simulink model "SolarMPPTController_New"  (R2019b)
settings: Solver=FixedStepAuto  StartTime=0.0  StopTime=6.0  RelTol=1e-3
libraries: powerlib x9, re_lib x1, powerlib_meascontrol x1, simulink x1
settings Model: Creator=DELL  LastModifiedBy=DELL

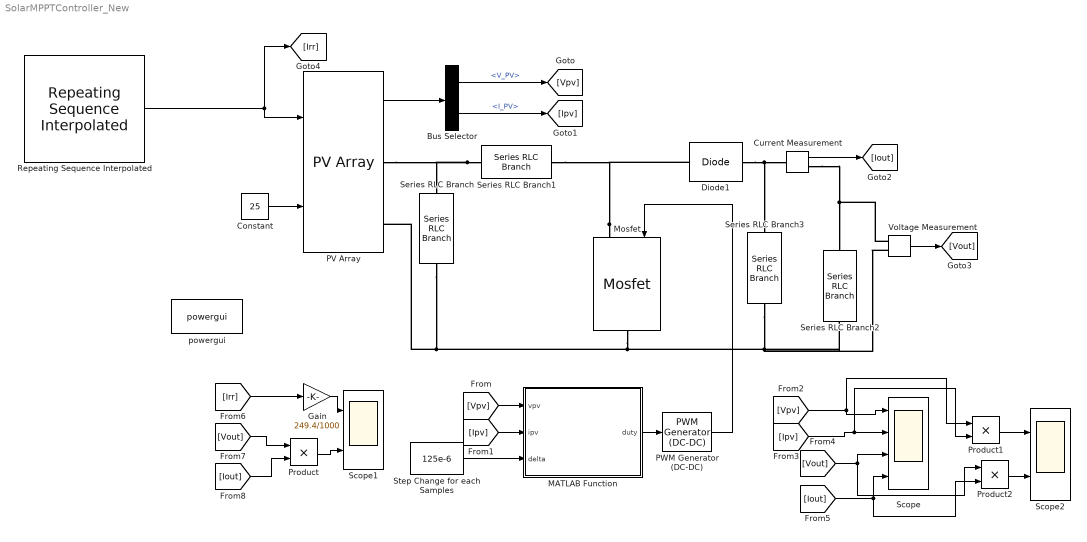
== system SolarMPPTController_New ==
  Bus Selector : BusSelector  OutputSignals=V_PV,I_PV
  Constant : Constant  Value=25
  Current Measurement : powerlib/Measurements/Current Measurement  PhasorSimulation=off  OutputType=Complex  PSBequivalent=0
      settings: SourceProductName=Simscape Electrical
  Diode1 : powerlib/Power Electronics/Diode  Ron=0.001  Lon=0  Vf=0.8  IC=0  UseSnubber=0  Rs=500  Cs=250e-9  Measurements=off
      settings: SourceProductName=Simscape Electrical
  Gain : Gain  Gain=249.4/1000
  MATLAB Function : MATLAB Function  TreatAsAtomicUnit=on
  Mosfet : powerlib/Power Electronics/Mosfet  Ron=0.1  Lon=0  Rd=0.01  Vfd=0  IC=0  Rs=1e5  Cs=inf  Measurements=off
      settings: SourceProductName=Simscape Electrical
  PV Array : re_lib/Solar/PV Array  Npar=1  Nser=1  PlotType=array @ 25 deg.C & specified irradiances  S_vec="[ 1000  500  100 ]"  Temp_C_vec="[ 45 25  ]"  ModuleName=1Soltech 1STH-FRL-4H-250-M60-BLK  PlotWhenSelected=off  Pm=248.977  Ncell=60  Voc=38.4  Isc=8.85  Vm=30.7  Im=8.11  beta_Voc_pc=-0.35599  alpha_Isc_pc=0.07  beta_Voc=-0.1367  alpha_Isc=0.006195  IL=8.8816  I0=2.622e-10  nI=1.0292  Rsh=104.8951  Rs=0.37421  BAL=off  Tc=1e-6  Tfilter=5e-5
      settings: SourceProductName=Simscape Electrical
  PWM Generator (DC-DC) : powerlib_meascontrol/Pulse & Signal Generators/PWM Generator (DC-DC)  Fsw=5000  Ts=1e-6
      settings: SourceProductName=Simscape Electrical
  Product : Product
  Product1 : Product
  Product2 : Product
  Repeating Sequence Interpolated : simulink/Sources/Repeating Sequence Interpolated  OutValues=[0 0 500 500 800 800 1000 1000 500 500 0 0]  TimeValues=[0 1.0 1.001 2.0 2.001 3.0 3.001 4.0 4.001 5.0 5.01 6.0]  LookUpMeth=Interpolation-Use End Values  tsamp=0.01  OutMin=[]  OutMax=[]  OutDataTypeStr=double  OutputDataTypeScalingMode=double  OutDataType=fixdt(0,8)  OutScaling=2^-10
  Scope : Scope  NumInputPorts=4
  Scope1 : Scope  NumInputPorts=2
  Scope2 : Scope  NumInputPorts=2
  Series RLC Branch : powerlib/Elements/Series RLC Branch  LConnTagsString=__new0  RConnTagsString=__new0  BranchType=C  Resistance=1e-6  Inductance=0  SetiL0=off  InitialCurrent=0  Capacitance=100e-6  Setx0=off  InitialVoltage=0  Measurements=None
      settings: SourceProductName=Simscape Electrical
  Series RLC Branch1 : powerlib/Elements/Series RLC Branch  LConnTagsString=__new0  RConnTagsString=__new0  BranchType=RL  Resistance=0.001  Inductance=900e-6  SetiL0=off  InitialCurrent=0  Capacitance=100e-6  Setx0=off  InitialVoltage=0  Measurements=None
      settings: SourceProductName=Simscape Electrical
  Series RLC Branch2 : powerlib/Elements/Series RLC Branch  LConnTagsString=__new0  RConnTagsString=__new0  BranchType=R  Resistance=20  Inductance=1e-3  SetiL0=off  InitialCurrent=0  Capacitance=100e-6  Setx0=off  InitialVoltage=0  Measurements=None
      settings: SourceProductName=Simscape Electrical
  Series RLC Branch3 : powerlib/Elements/Series RLC Branch  LConnTagsString=__new0  RConnTagsString=__new0  BranchType=C  Resistance=1e-6  Inductance=0  SetiL0=off  InitialCurrent=0  Capacitance=813e-6  Setx0=off  InitialVoltage=0  Measurements=None
      settings: SourceProductName=Simscape Electrical
  Step Change for each Samples : Constant  Value=125e-6
  Voltage Measurement : powerlib/Measurements/Voltage Measurement  PhasorSimulation=off  OutputType=Complex  PSBequivalent=0
      settings: SourceProductName=Simscape Electrical
  powergui : powerlib/powergui  Priority=1  SimulationMode=Discrete  SampleTime=5e-6  frequency=60  Iterations=50  frequencyindice=0  Pbase=100e6  ErrMax=1e-4  UnitsV=kV  UnitsW=MW  buscounter=0  FunctionMessages=off  echomessages=off  EnableUseOfTLC=off  CurrentSourceSwitches=off  DisableSnubberDevices=off  DisableRonSwitches=off  DisableVfSwitches=off  DisplayEquations=off  AutomaticDiscreteSolvers=off  SolverType=Tustin/Backward Euler (TBE)  Interpol=off  ExternalGateDelay=off  methode=off  Ts=100  x0status=blocks  SPID=on  SwTol=0  HookPort=off  NonlinearTolerance=1e-4  nMaxIteration=100  ContinueOnMaxIteration=off  RestoreLinks=warning  ResistiveCurrentMeasurement=off  Frange=[0:2:500]  Ylog=off  Xlog=on  ShowGrid=off  save=off  variable=ZData  structure=0  ZoomFFT=off  StartTime=0.0  cycles=1  DisplayStyle=1  fundamental=60  FreqAxis=off  MaxFrequency=1000  frequencyindicesteady=1  RmsSteady=1  display=off
      settings: SourceProductName=Simscape Electrical
  wires:
  Voltage Measurement/1 -> [Vout]
  [Ipv] -> Product1/2, Scope/2
  Step Change for each Samples/1 -> MATLAB Function/3(delta)
  [Vpv] -> Product1/1, Scope/1
  [Ipv] -> MATLAB Function/2(ipv)
  [Iout] -> Scope/4, Product2/2
  PV Array/1 -> Bus Selector/1
  MATLAB Function/1(duty) -> PWM Generator (DC-DC)/1
  PWM Generator (DC-DC)/1 -> Mosfet/1
  Bus Selector/2 -> [Ipv]  "<I_PV>"
  [Vpv] -> MATLAB Function/1(vpv)
  Bus Selector/1 -> [Vpv]  "<V_PV>"
  Constant/1 -> PV Array/2
  [Vout] -> Scope/3, Product2/1
  Current Measurement/1 -> [Iout]
  Repeating Sequence Interpolated/1 -> PV Array/1, [Irr]
  [Irr] -> Gain/1
  Gain/1 -> Scope1/1
  [Iout] -> Product/2
  [Vout] -> Product/1
  Product/1 -> Scope1/2
  Product1/1 -> Scope2/1
  Product2/1 -> Scope2/2
  connections:
  Series RLC Branch3/RConn1 -- Voltage Measurement/LConn2 -- Series RLC Branch2/LConn1 -- PV Array/RConn2 -- Series RLC Branch/RConn1 -- Mosfet/RConn1
  Series RLC Branch1/RConn1 -- PV Array/RConn1 -- Series RLC Branch/LConn1
  Mosfet/LConn1 -- Diode1/LConn1 -- Series RLC Branch1/LConn1
  Diode1/RConn1 -- Series RLC Branch3/LConn1 -- Current Measurement/LConn1
  Current Measurement/RConn1 -- Series RLC Branch2/RConn1 -- Voltage Measurement/LConn1

== matlab function SolarMPPTController_New/MATLAB Function ==
  data: vpv input; duty output; ipv input; delta input
function duty = MPPT_algorithm(vpv,ipv,delta)
duty_init = 0.1;
% min and max value are used to limit duty between
% 0 and 0.85
duty_min=0;
duty_max=0.85;

persistent Vold Pold duty_old;
% persistent variable type can be store the data
% we need the old data by obtain difference
% between old and new value
if isempty(Vold)
    Vold=0;
    Pold=0;
    duty_old=duty_init;
end
P= vpv*ipv; % power
dV= vpv - Vold; % difference between old and new voltage
dP= P - Pold;% difference between old and new power

% the algorithm in below search the dP/dV=0
% if the derivative equal to zero
% duty will not change
% if old and new power not equal
% &
% pv voltage bigger than 30V
% the algorithm will works
if dP ~= 0 && vpv>30
    if dP < 0
        if dV < 0
            duty = duty_old - delta;
        else
            duty = duty_old + delta;
        end
    else
        if dV < 0
            duty = duty_old + delta;
        else
            duty = duty_old - delta;
        end
    end
else
    duty = duty_old;
end

%the below if limits the duty between min and max
if duty >= duty_max
    duty=duty_max;
elseif duty<duty_min
    duty=duty_min;
end

% stored data
duty_old=duty;
Vold=vpv;
Pold=P;
